simulink model "Controllo_assex_4gdl"  (R2020b)
settings: Solver=VariableStepAuto  StartTime=0.0  StopTime=3  RelTol=1e-3
values from neighbouring files (symbols this model uses):
  m = config_dc(parx)    [main.m]
  parx = parametri()    [main.m]
undefined symbols (not defined in the file or in its folder): accelerazioni, Evaluate_Trajectory
libraries: cstblocks x10
settings Model: Creator=stefa  LastModifiedBy=user
settings DebuggingCC: SFMachineParentedDataDiag=error

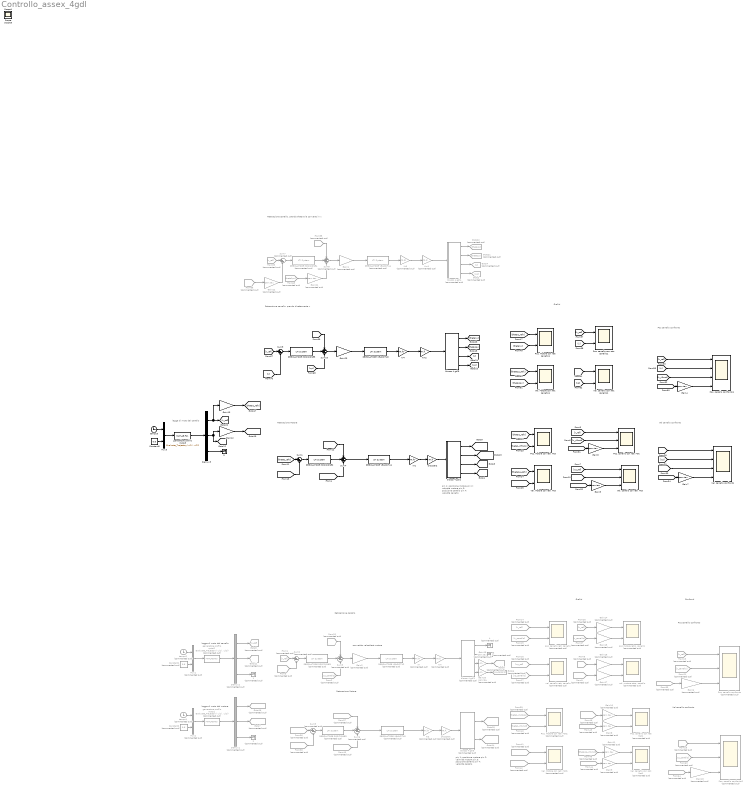
== system Controllo_assex_4gdl ==
  note: convertito velcotitaà motore
  note: pin 1: posizione motore
      | pin 2: velocità motore
      | pin 3: posizione carrello
      | pin 4: velocità carrello
  note: legge di moto del carrello
  note: Retroazione carrello
  note: Retroazione Motore
  note: Grafici
  note: Pos carrello confronto
  note: Vel carrello confronto
  note: legge di moto del motore
  note: pin 1: posizione motore
      | pin 2: velocità motore
      | pin 3: posizione carrello
      | pin 4: velocità carrello
  note: Retroazione Motore
  note: legge di moto del carrello
  note: Retroazione carrello, prendo theta e la converto in x
  note: Grafici
  note: Pos carrello confronto
  note: Confronti
  note: Vel carrello confronto
  note: Retroazione carrello, prendo direttamente x
   {1..2,4..5} (4 alike) : Terminator  Commented=on
  " 3" : Terminator
  Constant1 : Constant  Commented=on  Value=0.6
  Constant2 : Constant  Commented=on  Value=0.6
  Constant3 : Constant  Value=0.6
  Demux1 : Demux  Commented=on  Outputs=3
  Demux2 : Demux  Commented=on  Outputs=3
  Demux3 : Demux  Outputs=3
  From{1,14,19,26,35} (5 alike) : From  Commented=on  GotoTag=x_ref
  From{3,15,21,27} (4 alike) : From  Commented=on  GotoTag=x_carrello
  From{8,16,18,20,55} (5 alike) : From  Commented=on  GotoTag=xp_ref
  From{2,9,17,63} (4 alike) : From  Commented=on  GotoTag=xp_carrello
  From{33,38..39,43} (4 alike) : From  Commented=on  GotoTag=theta1_motore
  From36 : From  Commented=on  GotoTag=theta1_rif_mot
  From37 : From  Commented=on  GotoTag=theta1p_rif_mot
  From40 : From  Commented=on  GotoTag=theta1_rif_mot
  From{41,44..45,64} (4 alike) : From  Commented=on  GotoTag=theta1p_motore
  From42 : From  Commented=on  GotoTag=theta1p_rif_mot
  From46 : From  Commented=on  GotoTag=theta1_rif_mot
  From48 : From  Commented=on  GotoTag=theta1p_rif_mot
  From65 : From  Commented=on  GotoTag=theta1px
  From66 : From  Commented=on  GotoTag=theta1px
  Gain{1..2,14..17} (6 alike) : Gain  Commented=on  Gain=1/parx.tau
  Gain{8..11,19..22} (8 alike) : Gain  Commented=on  Gain=parx.tau
  Gain12 : Gain  Gain=1/parx.tau
  Gain13 : Gain  Gain=1/parx.tau
  Gain18 : Gain  Commented=on  Gain=(parx.tau)*178
  Gain23 : Gain  Gain=1/parx.tau
  Gain{3..5,7} (4 alike) : Gain  Gain=parx.tau
  Gain6 : Gain  Commented=on  Gain=(parx.tau)*178
  Goto11 : Goto  Commented=on  GotoTag=xp_ref
  Goto14 : Goto  Commented=on  GotoTag=theta1p_motore
  Goto16 : Goto  Commented=on  GotoTag=theta1_rif_mot
  Goto18 : Goto  Commented=on  GotoTag=theta1_motore
  Goto2 : Goto  Commented=on  GotoTag=xp
  Goto21 : Goto  Commented=on  GotoTag=theta1px
  Goto22 : Goto  Commented=on  GotoTag=theta1x
  Goto4 : Goto  Commented=on  GotoTag=x
  Goto5 : Goto  Commented=on  GotoTag=x_carrello
  Goto6 : Goto  Commented=on  GotoTag=xp_carrello
  Goto7 : Goto  Commented=on  GotoTag=theta1p_rif_mot
  Goto8 : Goto  Commented=on  GotoTag=x_ref
  Km : Gain  Commented=on  Gain=m.K
  Km1 : Gain  Commented=on  Gain=m.K
  Km2 : Gain  Gain=m.K
  Kr : Gain  Commented=on  Gain=m.kr
  Kr1 : Gain  Gain=m.kr
  Kr2 : Gain  Commented=on  Gain=m.kr
  Kr3 : Gain  Commented=on  Gain=m.kr
  Kr4 : Gain  Gain=m.kr
  Mux1 : Mux  Commented=on  Inputs=2
  Mux2 : Mux  Commented=on  Inputs=2
  Mux3 : Mux  Inputs=2
  Pos. Motore con retr. Mot : Scope  NumInputPorts=2
  Pos. Motore con retr. Mot1 : Scope  Commented=on  NumInputPorts=2
  Pos. Motore con retr. carrello1 : Scope  NumInputPorts=2
  Pos. carrello con retr. Mot : Scope  NumInputPorts=3
  Pos. carrello con retr. Mot1 : Scope  Commented=on  NumInputPorts=2
  Pos. carrello con retr. carrello1 : Scope  NumInputPorts=2
  Pos. carrello confronto : Scope  Commented=on  NumInputPorts=3
  Pos. carrello confronto1 : Scope  NumInputPorts=4
  Pos. carrello confronto2 : Scope  Commented=on  NumInputPorts=3
  REGOLATORE POSIZIONE1 : cstblocks/LTI System  Commented=on  sys=ap.H_P  IC=[]
  REGOLATORE POSIZIONE2 : cstblocks/LTI System  sys=ap.H_P  IC=[]
  REGOLATORE POSIZIONE3 : cstblocks/LTI System  Commented=on  sys=ap.H_P  IC=[]
  REGOLATORE POSIZIONE4 : cstblocks/LTI System  Commented=on  sys=ap.H_P  IC=[]
  REGOLATORE POSIZIONE5 : cstblocks/LTI System  sys=ap.H_P  IC=[]
  REGOLATORE VELOCITA1 : cstblocks/LTI System  sys=av.PI_V  IC=[]
  REGOLATORE VELOCITA2 : cstblocks/LTI System  Commented=on  sys=av.PI_V  IC=[]
  REGOLATORE VELOCITA3 : cstblocks/LTI System  Commented=on  sys=av.PI_V  IC=[]
  REGOLATORE VELOCITA4 : cstblocks/LTI System  Commented=on  sys=av.PI_V  IC=[]
  REGOLATORE VELOCITA5 : cstblocks/LTI System  sys=av.PI_V  IC=[]
  Sum1 : Sum  Inputs=|+-
  Sum10 : Sum  Inputs=++-
  Sum2 : Sum  Commented=on  Inputs=|+-
  Sum3 : Sum  Commented=on  Inputs=++-
  Sum4 : Sum  Inputs=++-
  Sum5 : Sum  Commented=on  Inputs=|+-
  Sum6 : Sum  Commented=on  Inputs=++-
  Sum7 : Sum  Commented=on  Inputs=|+-
  Sum8 : Sum  Commented=on  Inputs=++-
  Sum9 : Sum  Inputs=|+-
  Vel. Motore con retr. Mot : Scope  NumInputPorts=2
  Vel. Motore con retr. Mot1 : Scope  Commented=on  NumInputPorts=2
  Vel. Motore con retr. carrello1 : Scope  NumInputPorts=2
  Vel. carrello con retr. Mot : Scope  NumInputPorts=3
  Vel. carrello con retr. Mot1 : Scope  Commented=on  NumInputPorts=2
  Vel. carrello con retr. carrello1 : Scope  NumInputPorts=2
  Vel. carrello confronto : Scope  NumInputPorts=4
  blocco 4 gdl1 : Subsystem  Commented=on
  blocco 4 gdl2 : Subsystem
  blocco 4 gdl3 : Subsystem  Commented=on
  blocco 4 gdl4 : Subsystem  Commented=on
  blocco 4 gdl5 : Subsystem
  chopper1 : Gain  Commented=on  Gain=m.K
  chopper2 : Gain  Gain=m.K
  generatore profilo moto1 : MATLABFcn  Commented=on  MATLABFcn=Evaluate_Trajectory( u(1) , u(2))  OutputDimensions=3
  generatore profilo moto2 : MATLABFcn  Commented=on  MATLABFcn=Evaluate_Trajectory( u(1) , u(2))  OutputDimensions=3
  generatore profilo moto3 : MATLABFcn  MATLABFcn=Evaluate_Trajectory( u(1) , u(2))  OutputDimensions=3
  pos motore retro. carrello : Scope  Commented=on  NumInputPorts=2
  pos. carrello retr. carrello : Scope  Commented=on  NumInputPorts=2
  tempo1 : Clock  Commented=on
  tempo2 : Clock  Commented=on
  tempo3 : Clock
  vel. carrello retr. carrello : Scope  Commented=on  NumInputPorts=2
  vel. motore retro. carrello : Scope  Commented=on  NumInputPorts=2
  Scope : Scope
  Scope1 : Scope
  Scope3 : Scope
  wires:
  Kr/1 -> Km/1  "I"
  REGOLATORE VELOCITA2/1 -> Kr/1  "Va"
  REGOLATORE POSIZIONE1/1 -> Sum3/2
  Demux2/3 -> " 1"/1  "XPP"
  Mux1/1 -> generatore profilo moto2/1
  generatore profilo moto2/1 -> Demux2/1  "carrello"
  Constant1/1 -> Mux1/2
  Sum2/1 -> REGOLATORE POSIZIONE1/1
  tempo2/1 -> Mux1/1
  Demux2/1 -> Goto8/1  "X"
  Demux2/2 -> Goto11/1  "XP"
  From20/1 -> Sum3/1
  Sum3/1 -> Gain2/1
  Gain2/1 -> REGOLATORE VELOCITA2/1  "theta1_rifx"
  From1/1 -> Sum2/1
  From3/1 -> Sum2/2
  From2/1 -> Sum3/3
  [x_rifmot] -> Pos. carrello con retr. Mot/2
  [theta1_refx] -> Pos. Motore con retr. Mot/1
  Kr1/1 -> chopper2/1  "I"
  Sum1/1 -> REGOLATORE POSIZIONE2/1
  [theta1p_refx] -> Vel. Motore con retr. Mot/1
  REGOLATORE POSIZIONE2/1 -> Sum4/2
  REGOLATORE VELOCITA1/1 -> Kr1/1  "Va"
  [xp_rifmot] -> Vel. carrello con retr. Mot/2
  [xp_ref] -> Vel. carrello con retr. Mot/1
  Sum4/1 -> REGOLATORE VELOCITA1/1
  [x_ref] -> Pos. carrello con retr. Mot/1
  [theta1p_rifmotx] -> Vel. Motore con retr. Mot/2
  [theta1_rifmotx] -> Pos. Motore con retr. Mot/2
  [theta1p_refx] -> Sum4/1
  [theta1_refx] -> Sum1/1
  [theta1p_rifmotx] -> Sum4/3
  [theta1_rifmotx] -> Sum1/2
  From17/1 -> vel. carrello retr. carrello/2  "x_carrello"
  From15/1 -> pos. carrello retr. carrello/2  "x_carrello"
  From16/1 -> vel. carrello retr. carrello/1  "rif_carrello"
  From14/1 -> pos. carrello retr. carrello/1  "rif_carrello"
  From21/1 -> Pos. carrello confronto/2  "posizione_carrello"
  From19/1 -> Pos. carrello confronto/1  "riferimento carrello"
  [xp] -> Vel. carrello confronto/2  "velocita_carrello"
  [xp_ref] -> Vel. carrello confronto/1  "riferimento carrello"
  [xp_rifmot] -> Vel. carrello confronto/3  "velocita_motore1"
  Km/1 -> blocco 4 gdl1/1(In1)  "Cm"
  chopper2/1 -> blocco 4 gdl2/1(In1)  "Cm"
  blocco 4 gdl1/1(Out7) -> " 4"/1
  blocco 4 gdl1/2(Out8) -> " 5"/1
  blocco 4 gdl2/1(Out3) -> [theta1_rifmotx]
  blocco 4 gdl2/3(Out7) -> [x_rifmot]
  blocco 4 gdl2/2(Out4) -> [theta1p_rifmotx]
  blocco 4 gdl2/4(Out1) -> [xp_rifmot]
  [theta1_rifmotx] -> Gain3/1
  Gain3/1 -> Pos. carrello con retr. Mot/3  "motore"
  Gain5/1 -> Vel. carrello con retr. Mot/3  "motore"
  [theta1p_rifmotx] -> Gain5/1
  From33/1 -> Gain6/1
  Gain6/1 -> Pos. carrello confronto/3  "posizione_motore"
  [theta1p_rifmotx] -> Gain7/1
  Gain7/1 -> Vel. carrello confronto/4  "velocita_motore2"
  generatore profilo moto1/1 -> Demux1/1  "motore"
  Constant2/1 -> Mux2/2
  Demux1/2 -> Goto7/1  "XP"
  Demux1/1 -> Goto16/1  "X"
  Demux1/3 -> " 2"/1  "XPP"
  tempo1/1 -> Mux2/1
  Mux2/1 -> generatore profilo moto1/1
  Gain9/1 -> Vel. carrello con retr. Mot1/2  "xp_carrello"
  From43/1 -> Gain8/1
  From44/1 -> Gain9/1
  REGOLATORE POSIZIONE3/1 -> Sum6/2
  blocco 4 gdl3/1(Out3) -> Goto18/1
  blocco 4 gdl3/2(Out4) -> Goto14/1
  From40/1 -> Pos. Motore con retr. Mot1/2  "x_motore"
  Sum6/1 -> REGOLATORE VELOCITA3/1
  From46/1 -> Gain10/1
  Gain8/1 -> Pos. carrello con retr. Mot1/2  "x_carrello"
  Kr2/1 -> chopper1/1  "I"
  chopper1/1 -> blocco 4 gdl3/1(In1)  "Cm"
  From45/1 -> Sum6/3
  From36/1 -> Sum5/1
  From38/1 -> Sum5/2
  From37/1 -> Sum6/1
  Sum5/1 -> REGOLATORE POSIZIONE3/1
  From42/1 -> Vel. Motore con retr. Mot1/2  "xp_motore"
  From39/1 -> Pos. Motore con retr. Mot1/1  "rif_mot"
  REGOLATORE VELOCITA3/1 -> Kr2/1  "Va"
  From41/1 -> Vel. Motore con retr. Mot1/1  "rif_mot"
  Gain10/1 -> Pos. carrello con retr. Mot1/1  "carrello_rif"
  From48/1 -> Gain11/1
  Gain11/1 -> Vel. carrello con retr. Mot1/1  "carrello_rif"
  generatore profilo moto3/1 -> Demux3/1  "carrello"
  Gain12/1 -> [theta1p_refx]  "motore"
  Gain13/1 -> [theta1_refx]  "motore"
  Constant3/1 -> Mux3/2
  Demux3/2 -> Gain12/1, [xp_ref]  "XP"
  Demux3/1 -> [x_ref], Gain13/1  "X"
  Demux3/3 -> " 3"/1  "XPP"
  tempo3/1 -> Mux3/1
  Mux3/1 -> generatore profilo moto3/1
  Gain4/1 -> Pos. carrello confronto1/4  "posizione_motore2"
  [theta1px] -> Vel. Motore con retr. carrello1/2
  [x] -> Pos. carrello confronto1/2  "posizione_carrello"
  [theta1_refx] -> Pos. Motore con retr. carrello1/1
  blocco 4 gdl4/4(Out8) -> Goto2/1
  Km1/1 -> blocco 4 gdl4/1(In1)  "Cm"
  blocco 4 gdl4/2(Out4) -> Goto21/1
  [theta1_rifmotx] -> Gain4/1
  blocco 4 gdl4/3(Out7) -> Goto4/1
  Sum7/1 -> REGOLATORE POSIZIONE4/1
  blocco 4 gdl4/1(Out3) -> Goto22/1
  [theta1p_refx] -> Vel. Motore con retr. carrello1/1
  [x_ref] -> Pos. carrello confronto1/1  "riferimento carrello"
  From35/1 -> Sum7/1
  [theta1x] -> Pos. Motore con retr. carrello1/2
  [xp] -> Vel. carrello con retr. carrello1/2
  [x_rifmot] -> Pos. carrello confronto1/3  "posizioine_motore1"
  From55/1 -> Sum8/1
  Sum8/1 -> Gain1/1
  [x] -> Pos. carrello con retr. carrello1/2
  [x_ref] -> Pos. carrello con retr. carrello1/1
  [xp_ref] -> Vel. carrello con retr. carrello1/1
  REGOLATORE POSIZIONE4/1 -> Sum8/2
  Kr3/1 -> Km1/1  "I"
  REGOLATORE VELOCITA4/1 -> Kr3/1  "Va"
  Gain1/1 -> REGOLATORE VELOCITA4/1  "theta1_rifx"
  Gain14/1 -> pos motore retro. carrello/1  "rif_mot"
  From26/1 -> Gain14/1
  From27/1 -> Gain15/1
  Gain15/1 -> pos motore retro. carrello/2  "x_carrello"
  Gain17/1 -> vel. motore retro. carrello/2  "xp_motore"
  From9/1 -> Gain17/1
  From8/1 -> Gain16/1
  Gain16/1 -> vel. motore retro. carrello/1  "rif_mot"
  From64/1 -> Gain18/1
  From18/1 -> Pos. carrello confronto2/1  "riferimento carrello"
  Gain18/1 -> Pos. carrello confronto2/3  "velocita_motore"
  From63/1 -> Pos. carrello confronto2/2  "velocita_carrello"
  blocco 4 gdl1/3(Out1) -> Gain19/1
  blocco 4 gdl1/4(Out2) -> Gain20/1
  Gain19/1 -> Goto5/1  "theta1_rifx"
  Gain20/1 -> Goto6/1  "theta1_rifx"
  From65/1 -> Gain21/1
  Gain21/1 -> Sum8/3  "theta1_rifx"
  From66/1 -> Gain22/1
  Gain22/1 -> Sum7/2  "theta1_rifx"
  [x] -> Sum9/2  "theta1_rifx"
  Gain23/1 -> REGOLATORE VELOCITA5/1  "theta1_rifx"
  blocco 4 gdl5/4(Out8) -> [xp]
  REGOLATORE VELOCITA5/1 -> Kr4/1  "Va"
  Km2/1 -> blocco 4 gdl5/1(In1)  "Cm"
  Sum10/1 -> Gain23/1
  blocco 4 gdl5/3(Out7) -> [x]
  REGOLATORE POSIZIONE5/1 -> Sum10/2
  [x_ref] -> Sum9/1
  blocco 4 gdl5/2(Out4) -> [theta1px]
  [xp_ref] -> Sum10/1
  Sum9/1 -> REGOLATORE POSIZIONE5/1
  [xp] -> Sum10/3  "theta1_rifx"
  Kr4/1 -> Km2/1  "I"
  blocco 4 gdl5/1(Out3) -> [theta1x]

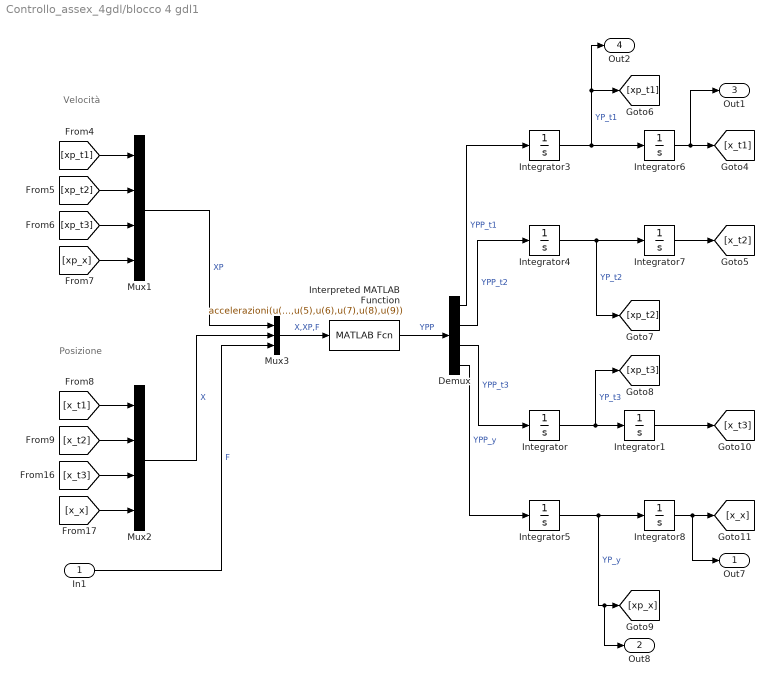
== system Controllo_assex_4gdl/blocco 4 gdl1 ==
  note: Velocità
  note: Posizione
  In1 : Inport
  Demux : Demux
  Integrator{,1,3..8} (8 alike) : Integrator
  Interpreted MATLAB Function : MATLABFcn  MATLABFcn=accelerazioni(u(1),u(2),u(3),u(4),u(5),u(6),u(7),u(8),u(9))  OutputDimensions=4
  Mux1 : Mux
  Mux2 : Mux
  Mux3 : Mux  Inputs=3
  Out7 : Outport
  Out8 : Outport  Port=2
  Out1 : Outport  Port=3
  Out2 : Outport  Port=4
  wires:
  Integrator4/1 -> [xp_t2], Integrator7/1  "YP_t2"
  [xp_t1] -> Mux1/1
  [x_t2] -> Mux2/2
  Integrator1/1 -> [x_t3]
  Demux/4 -> Integrator5/1  "YPP_y"
  Demux/2 -> Integrator4/1  "YPP_t2"
  In1/1 -> Mux3/3  "F"
  Mux3/1 -> Interpreted MATLAB Function/1  "X,XP,F"
  [xp_t2] -> Mux1/2
  Integrator6/1 -> Out1/1, [x_t1]
  Mux2/1 -> Mux3/2  "X"
  Demux/3 -> Integrator/1  "YPP_t3"
  Integrator5/1 -> Out8/1, [xp_x], Integrator8/1  "YP_y"
  Integrator8/1 -> Out7/1, [x_x]
  [xp_x] -> Mux1/4
  [x_x] -> Mux2/4
  Integrator7/1 -> [x_t2]
  Demux/1 -> Integrator3/1  "YPP_t1"
  [x_t1] -> Mux2/1
  Integrator3/1 -> Out2/1, [xp_t1], Integrator6/1  "YP_t1"
  [x_t3] -> Mux2/3
  Interpreted MATLAB Function/1 -> Demux/1  "YPP"
  Mux1/1 -> Mux3/1  "XP"
  Integrator/1 -> Integrator1/1, [xp_t3]  "YP_t3"
  [xp_t3] -> Mux1/3

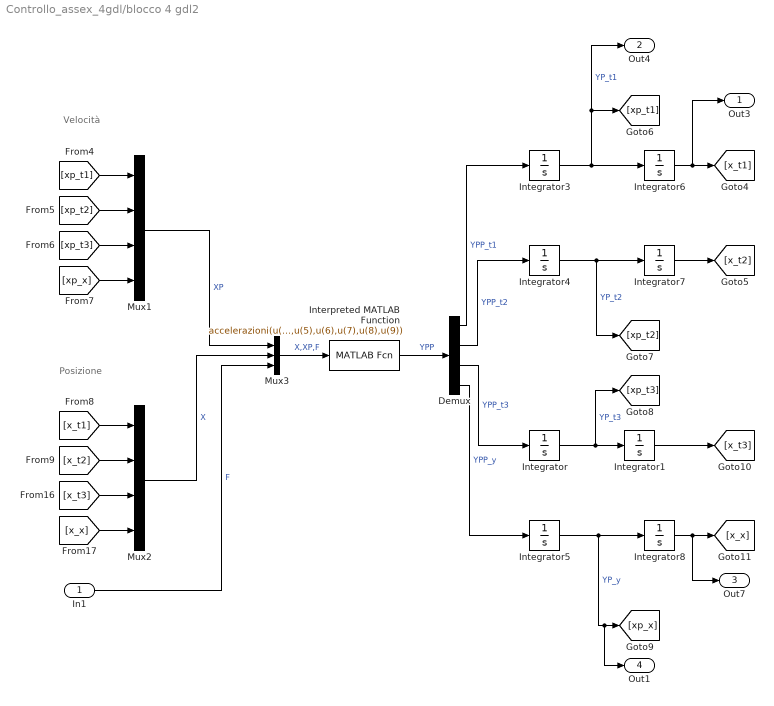
== system Controllo_assex_4gdl/blocco 4 gdl2 ==
  note: Posizione
  note: Velocità
  In1 : Inport
  Demux : Demux
  Integrator{,1,3..7} (7 alike) : Integrator
  Integrator8 : Integrator  InitialCondition=0.0005
  Interpreted MATLAB Function : MATLABFcn  MATLABFcn=accelerazioni(u(1),u(2),u(3),u(4),u(5),u(6),u(7),u(8),u(9))  OutputDimensions=4
  Mux1 : Mux
  Mux2 : Mux
  Mux3 : Mux  Inputs=3
  Out3 : Outport
  Out4 : Outport  Port=2
  Out7 : Outport  Port=3
  Out1 : Outport  Port=4
  wires:
  [xp_t3] -> Mux1/3
  Interpreted MATLAB Function/1 -> Demux/1  "YPP"
  Integrator3/1 -> Out4/1, [xp_t1], Integrator6/1  "YP_t1"
  Integrator8/1 -> Out7/1, [x_x]
  Integrator7/1 -> [x_t2]
  [xp_x] -> Mux1/4
  [x_t1] -> Mux2/1
  Mux1/1 -> Mux3/1  "XP"
  [x_x] -> Mux2/4
  Demux/3 -> Integrator/1  "YPP_t3"
  Integrator/1 -> Integrator1/1, [xp_t3]  "YP_t3"
  Mux2/1 -> Mux3/2  "X"
  Integrator6/1 -> Out3/1, [x_t1]
  Integrator5/1 -> Out1/1, [xp_x], Integrator8/1  "YP_y"
  [xp_t2] -> Mux1/2
  Mux3/1 -> Interpreted MATLAB Function/1  "X,XP,F"
  [x_t3] -> Mux2/3
  In1/1 -> Mux3/3  "F"
  Demux/4 -> Integrator5/1  "YPP_y"
  Integrator4/1 -> [xp_t2], Integrator7/1  "YP_t2"
  Integrator1/1 -> [x_t3]
  [xp_t1] -> Mux1/1
  [x_t2] -> Mux2/2
  Demux/2 -> Integrator4/1  "YPP_t2"
  Demux/1 -> Integrator3/1  "YPP_t1"

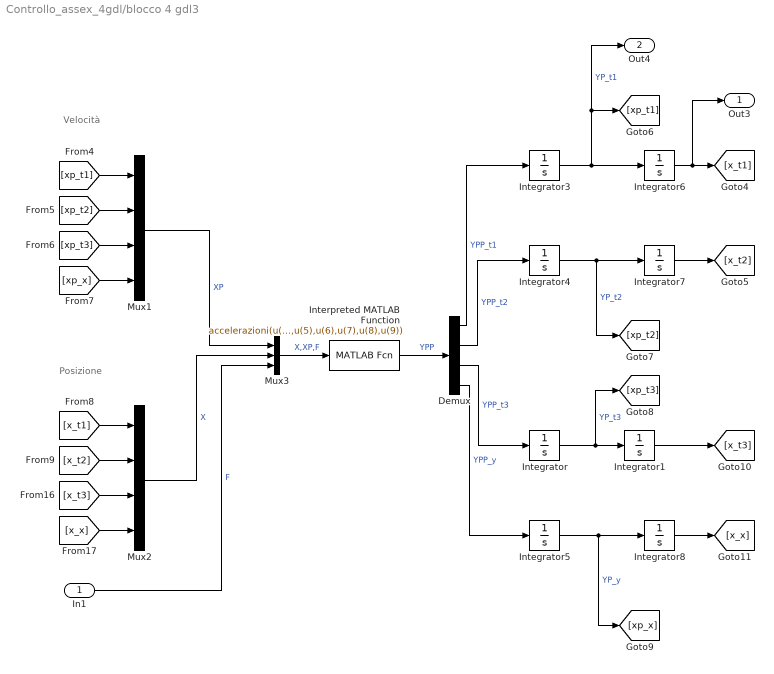
== system Controllo_assex_4gdl/blocco 4 gdl3 ==
  note: Posizione
  note: Velocità
  In1 : Inport
  Demux : Demux
  Integrator{,1,3..8} (8 alike) : Integrator
  Interpreted MATLAB Function : MATLABFcn  MATLABFcn=accelerazioni(u(1),u(2),u(3),u(4),u(5),u(6),u(7),u(8),u(9))  OutputDimensions=4
  Mux1 : Mux
  Mux2 : Mux
  Mux3 : Mux  Inputs=3
  Out3 : Outport
  Out4 : Outport  Port=2
  wires:
  [xp_t3] -> Mux1/3
  Interpreted MATLAB Function/1 -> Demux/1  "YPP"
  Integrator3/1 -> Out4/1, [xp_t1], Integrator6/1  "YP_t1"
  Integrator8/1 -> [x_x]
  Integrator7/1 -> [x_t2]
  [xp_x] -> Mux1/4
  [x_t1] -> Mux2/1
  Mux1/1 -> Mux3/1  "XP"
  [x_x] -> Mux2/4
  Demux/3 -> Integrator/1  "YPP_t3"
  Integrator/1 -> Integrator1/1, [xp_t3]  "YP_t3"
  Mux2/1 -> Mux3/2  "X"
  Integrator6/1 -> Out3/1, [x_t1]
  Integrator5/1 -> [xp_x], Integrator8/1  "YP_y"
  [xp_t2] -> Mux1/2
  Mux3/1 -> Interpreted MATLAB Function/1  "X,XP,F"
  [x_t3] -> Mux2/3
  In1/1 -> Mux3/3  "F"
  Demux/4 -> Integrator5/1  "YPP_y"
  Integrator4/1 -> [xp_t2], Integrator7/1  "YP_t2"
  Integrator1/1 -> [x_t3]
  [xp_t1] -> Mux1/1
  [x_t2] -> Mux2/2
  Demux/2 -> Integrator4/1  "YPP_t2"
  Demux/1 -> Integrator3/1  "YPP_t1"

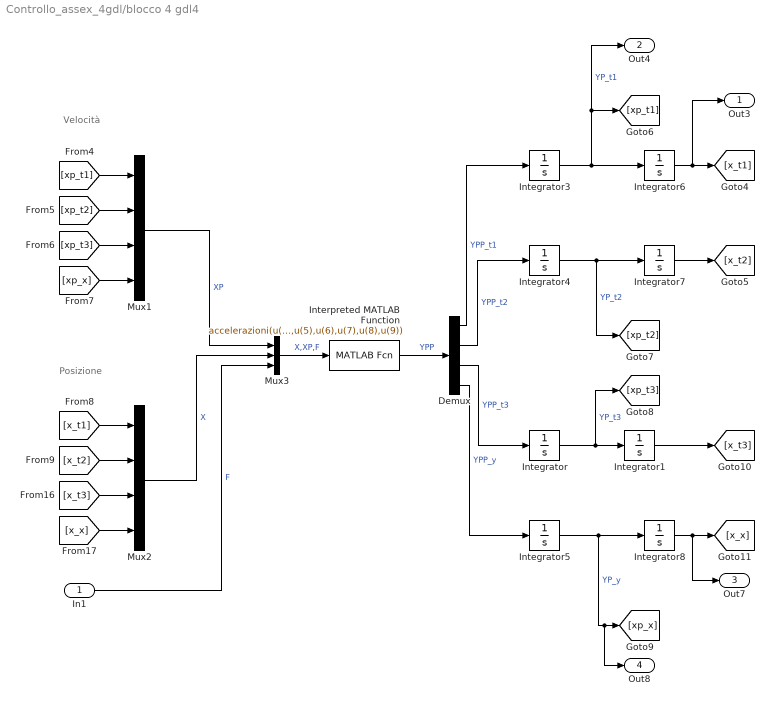
== system Controllo_assex_4gdl/blocco 4 gdl4 ==
  note: Velocità
  note: Posizione
  In1 : Inport
  Demux : Demux
  Integrator{,1,3..7} (7 alike) : Integrator
  Integrator8 : Integrator  InitialCondition=0.0005
  Interpreted MATLAB Function : MATLABFcn  MATLABFcn=accelerazioni(u(1),u(2),u(3),u(4),u(5),u(6),u(7),u(8),u(9))  OutputDimensions=4
  Mux1 : Mux
  Mux2 : Mux
  Mux3 : Mux  Inputs=3
  Out3 : Outport
  Out4 : Outport  Port=2
  Out7 : Outport  Port=3
  Out8 : Outport  Port=4
  wires:
  Integrator4/1 -> [xp_t2], Integrator7/1  "YP_t2"
  [xp_t1] -> Mux1/1
  [x_t2] -> Mux2/2
  Integrator1/1 -> [x_t3]
  Demux/4 -> Integrator5/1  "YPP_y"
  Demux/2 -> Integrator4/1  "YPP_t2"
  In1/1 -> Mux3/3  "F"
  Mux3/1 -> Interpreted MATLAB Function/1  "X,XP,F"
  [xp_t2] -> Mux1/2
  Integrator6/1 -> Out3/1, [x_t1]
  Mux2/1 -> Mux3/2  "X"
  Demux/3 -> Integrator/1  "YPP_t3"
  Integrator5/1 -> Out8/1, [xp_x], Integrator8/1  "YP_y"
  Integrator8/1 -> Out7/1, [x_x]
  [xp_x] -> Mux1/4
  [x_x] -> Mux2/4
  Integrator7/1 -> [x_t2]
  Demux/1 -> Integrator3/1  "YPP_t1"
  [x_t1] -> Mux2/1
  Integrator3/1 -> Out4/1, [xp_t1], Integrator6/1  "YP_t1"
  [x_t3] -> Mux2/3
  Interpreted MATLAB Function/1 -> Demux/1  "YPP"
  Mux1/1 -> Mux3/1  "XP"
  Integrator/1 -> Integrator1/1, [xp_t3]  "YP_t3"
  [xp_t3] -> Mux1/3

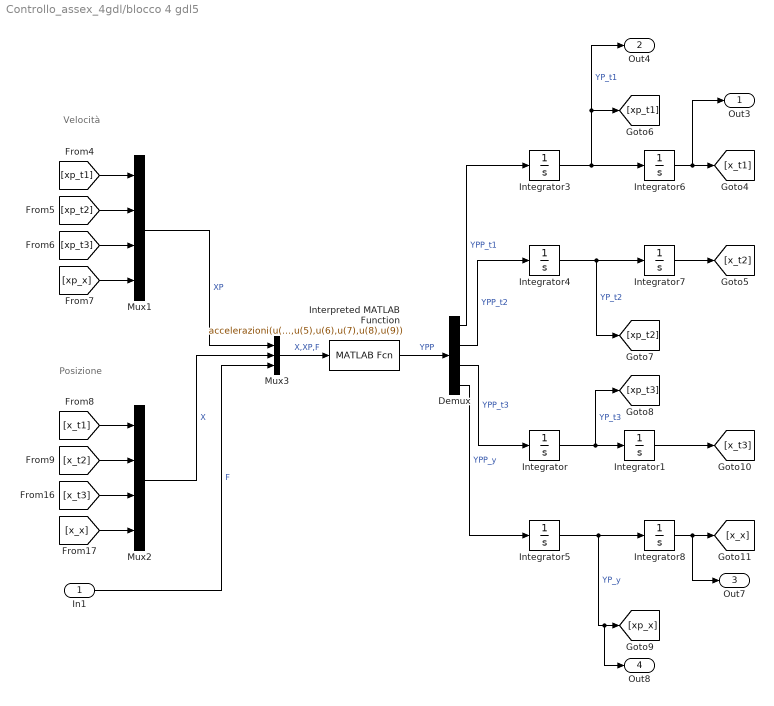
== system Controllo_assex_4gdl/blocco 4 gdl5 ==
  note: Velocità
  note: Posizione
  In1 : Inport
  Demux : Demux
  Integrator{,1,3..7} (7 alike) : Integrator
  Integrator8 : Integrator  InitialCondition=0.0005
  Interpreted MATLAB Function : MATLABFcn  MATLABFcn=accelerazioni(u(1),u(2),u(3),u(4),u(5),u(6),u(7),u(8),u(9))  OutputDimensions=4
  Mux1 : Mux
  Mux2 : Mux
  Mux3 : Mux  Inputs=3
  Out3 : Outport
  Out4 : Outport  Port=2
  Out7 : Outport  Port=3
  Out8 : Outport  Port=4
  wires:
  Integrator4/1 -> [xp_t2], Integrator7/1  "YP_t2"
  [xp_t1] -> Mux1/1
  [x_t2] -> Mux2/2
  Integrator1/1 -> [x_t3]
  Demux/4 -> Integrator5/1  "YPP_y"
  Demux/2 -> Integrator4/1  "YPP_t2"
  In1/1 -> Mux3/3  "F"
  Mux3/1 -> Interpreted MATLAB Function/1  "X,XP,F"
  [xp_t2] -> Mux1/2
  Integrator6/1 -> Out3/1, [x_t1]
  Mux2/1 -> Mux3/2  "X"
  Demux/3 -> Integrator/1  "YPP_t3"
  Integrator5/1 -> Out8/1, [xp_x], Integrator8/1  "YP_y"
  Integrator8/1 -> Out7/1, [x_x]
  [xp_x] -> Mux1/4
  [x_x] -> Mux2/4
  Integrator7/1 -> [x_t2]
  Demux/1 -> Integrator3/1  "YPP_t1"
  [x_t1] -> Mux2/1
  Integrator3/1 -> Out4/1, [xp_t1], Integrator6/1  "YP_t1"
  [x_t3] -> Mux2/3
  Interpreted MATLAB Function/1 -> Demux/1  "YPP"
  Mux1/1 -> Mux3/1  "XP"
  Integrator/1 -> Integrator1/1, [xp_t3]  "YP_t3"
  [xp_t3] -> Mux1/3
